simulink model "Logic_and_Bit_Operations_Lib"  (R2020b)
settings: Solver=VariableStepAuto  StartTime=0.0  StopTime=10.0  RelTol=1e-3
libraries: simulink x3
settings Model: Creator=Emiliano  LastModifiedBy=Emiliano
settings OptimizationCC: DefaultParameterBehavior=Inlined  UseDivisionForNetSlopeComputation=on  GainParamInheritBuiltInType=on  UseFloatMulNetSlope=on  InlineInvariantSignals=on  PassReuseOutputArgsAs=Individual arguments  ZeroExternalMemoryAtStartup=off  ZeroInternalMemoryAtStartup=off  NoFixptDivByZeroProtection=on  EfficientFloat2IntCast=on  LifeSpan=1  OptimizeBlockOrder=speed  DifferentSizesBufferReuse=on  EfficientTunableParamExpr=on
settings DebuggingCC: ParameterTunabilityLossMsg=error
settings HardwareCC: ProdLongLongMode=on
settings SFSimCC: MATLABDynamicMemAlloc=off
settings RTWCC: Description=Embedded Coder  SystemTargetFile=ert.tlc  TemplateMakefile=ert_default_tmf
settings CodeAppCC: ForceParamTrailComments=on  IgnoreCustomStorageClasses=off  OperatorAnnotations=on  SimulinkDataObjDesc=on  SFDataObjDesc=on  CustomSymbolStrGlobalVar=rt$N$M  CustomSymbolStrType=$N$M  CustomSymbolStrFcn=$N$M$F  CustomSymbolStrMacro=$N$M  InsertBlockDesc=on
settings ERTTargetCC: TargetLangStandard=C99 (ISO)  GenerateSampleERTMain=on  IncludeMdlTerminateFcn=off  CombineSignalStateStructs=on  SupportAbsoluteTime=off  SupportComplex=off  SupportContinuousTime=on  SupportNonInlinedSFcns=on  InlinedParameterPlacement=NonHierarchical  ERTCustomFileTemplate=example_file_process.tlc  ERTFilePackagingFormat=CompactWithDataFile

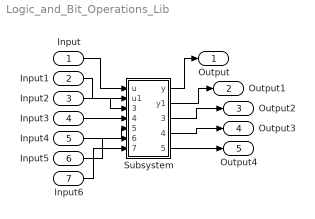
== system Logic_and_Bit_Operations_Lib ==
  Input : Inport
  Input1 : Inport  Port=2
  Input2 : Inport  Port=3
  Input3 : Inport  Port=4
  Input4 : Inport  Port=5
  Input5 : Inport  Port=6
  Input6 : Inport  Port=7
  Subsystem : Subsystem
  Output : Outport
  Output1 : Outport  Port=2
  Output2 : Outport  Port=3
  Output3 : Outport  Port=4
  Output4 : Outport  Port=5
  wires:
  Input/1 -> Subsystem/1(u)
  Input1/1 -> Subsystem/2(u1)
  Input2/1 -> Subsystem/3(In3)
  Input3/1 -> Subsystem/4(In4)
  Subsystem/1(y) -> Output/1
  Subsystem/2(y1) -> Output1/1
  Subsystem/3(Out3) -> Output2/1
  Input4/1 -> Subsystem/5(Input4)
  Input5/1 -> Subsystem/6(Input5)
  Input6/1 -> Subsystem/7(Input6)
  Subsystem/5(Output4) -> Output4/1
  Subsystem/4(Output3) -> Output3/1

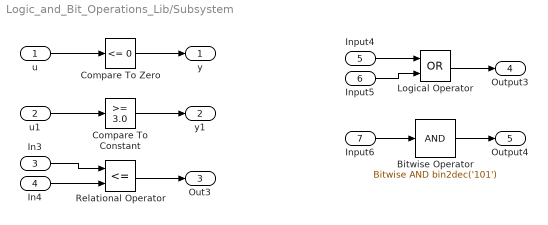
== system Logic_and_Bit_Operations_Lib/Subsystem ==
  u : Inport
  u1 : Inport  Port=2
  In3 : Inport  Port=3
  In4 : Inport  Port=4
  Input4 : Inport  Port=5
  Input5 : Inport  Port=6
  Input6 : Inport  Port=7  OutDataTypeStr=uint64
  Bitwise Operator : simulink/Logic and Bit Operations/Bitwise Operator  logicop=AND  UseBitMask=on  BitMask=bin2dec('101')  BitMaskRealWorld=Stored Integer
  Compare To Constant : simulink/Logic and Bit Operations/Compare To Constant  relop=>=  const=3.0  OutDataTypeStr=boolean
  Compare To Zero : simulink/Logic and Bit Operations/Compare To Zero  relop=<=  OutDataTypeStr=boolean
  Logical Operator : Logic  Operator=OR  AllPortsSameDT=off  OutDataTypeStr=boolean
  Relational Operator : RelationalOperator  Operator=<=  OutDataTypeStr=boolean  RndMeth=Simplest
  y : Outport
  y1 : Outport  Port=2
  Out3 : Outport  Port=3
  Output3 : Outport  Port=4
  Output4 : Outport  Port=5  OutDataTypeStr=uint64
  wires:
  u/1 -> Compare To Zero/1
  Relational Operator/1 -> Out3/1
  Compare To Constant/1 -> y1/1
  Compare To Zero/1 -> y/1
  In3/1 -> Relational Operator/1
  u1/1 -> Compare To Constant/1
  In4/1 -> Relational Operator/2
  Input4/1 -> Logical Operator/1
  Input5/1 -> Logical Operator/2
  Logical Operator/1 -> Output3/1
  Input6/1 -> Bitwise Operator/1
  Bitwise Operator/1 -> Output4/1
